simulink model "Inv_pendulum_cart_plant"  (R2022a)
settings: Solver=VariableStepAuto  StartTime=0.0  StopTime=10.0  RelTol=1e-3
values from neighbouring files (symbols this model uses):
  b = 0.02    [pendulum_cart.m]    (also in pendulum_cart_integral.m)
  g = 9.81    [pendulum_cart.m]    (also in pendulum_cart_integral.m)
  kv = 0.02    [pendulum_cart.m]    (also in pendulum_cart_integral.m)
  L = 1.0    (= 1)    [pendulum_cart.m]    (also in pendulum_cart_integral.m)
  M = 6.0    (= 6)    [pendulum_cart.m]    (also in pendulum_cart_integral.m)
  m = 1.5    [pendulum_cart.m]    (also in pendulum_cart_integral.m)
settings Model: Creator=Admin  LastModifiedBy=Admin

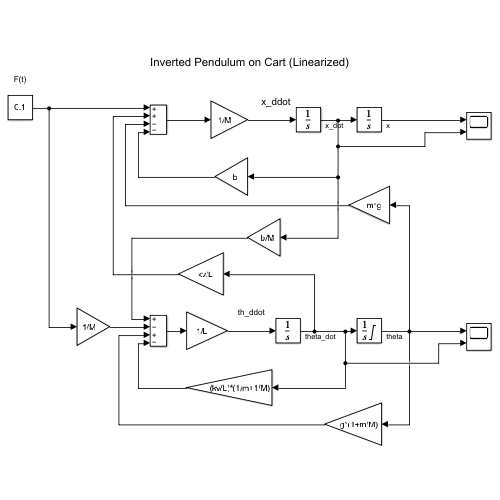
[thumbnail: Simulink's stored preview of the top-level diagram]
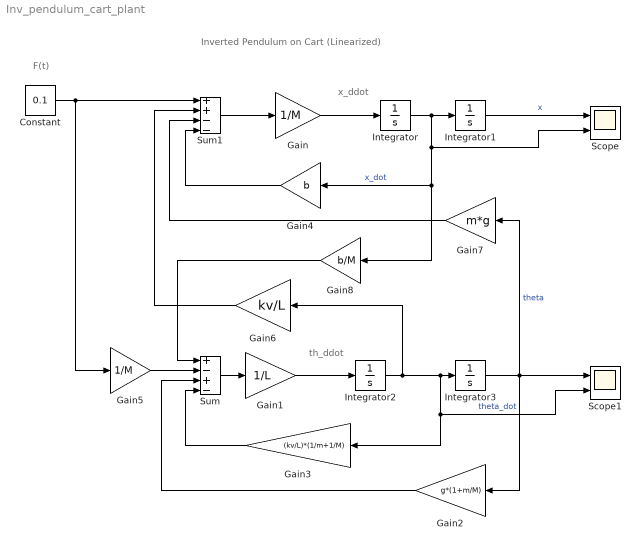
== system Inv_pendulum_cart_plant ==
  note: Inverted Pendulum on Cart (Linearized)
  note: F(t)
  note: x_ddot
  note: th_ddot
  Constant : Constant  Value=0.1
  Gain : Gain  Gain=1/M
  Gain1 : Gain  Gain=1/L
  Gain2 : Gain  Gain=g*(1+m/M)
  Gain3 : Gain  Gain=(kv/L)*(1/m+1/M)
  Gain4 : Gain  Gain=b
  Gain5 : Gain  Gain=1/M
  Gain6 : Gain  Gain=kv/L
  Gain7 : Gain  Gain=m*g
  Gain8 : Gain  Gain=b/M
  Integrator : Integrator
  Integrator1 : Integrator
  Integrator2 : Integrator
  Integrator3 : Integrator  LimitOutput=on  UpperSaturationLimit=+1.1*pi  LowerSaturationLimit=-1.1*pi
  Scope : Scope  NumInputPorts=2
  Scope1 : Scope  NumInputPorts=2
  Sum : Sum  Inputs=+-+-
  Sum1 : Sum  Inputs=++--
  wires:
  Gain/1 -> Integrator/1
  Integrator/1 -> Scope/2, Gain8/1, Gain4/1, Integrator1/1  "x_dot"
  Integrator2/1 -> Gain6/1, Gain3/1, Scope1/2, Integrator3/1  "theta_dot"
  Gain1/1 -> Integrator2/1
  Integrator3/1 -> Gain2/1, Gain7/1, Scope1/1  "theta"
  Sum/1 -> Gain1/1
  Sum1/1 -> Gain/1
  Constant/1 -> Gain5/1, Sum1/1
  Integrator1/1 -> Scope/1  "x"
  Gain4/1 -> Sum1/4
  Gain3/1 -> Sum/4
  Gain2/1 -> Sum/3
  Gain7/1 -> Sum1/3
  Gain6/1 -> Sum1/2
  Gain5/1 -> Sum/2
  Gain8/1 -> Sum/1
